simulink library "PowerFlowLib"  (R2016a)
settings: Solver=ode45  StartTime=0.0  StopTime=10.0  RelTol=1e-3
undefined symbols (not defined in the file or in its folder): Air, AirProp, C, F1, F2, Fanmap, Fld1, Fld2, Fluid, fueltankdata, HydProp, HydraulicLoad, IBFD_exc, L, LoadFluidProps, magnitude, MSSN, n_alghts, PumpProp, pwr_alghts, R_fd_exc, Rcore, Ts, VBFD_exc
libraries: PowerFlowLib x35, simulink x19, powerlib_extras x2, dspstat3 x2
(part 11 of 12)

== system PowerFlowLib/Energy & Power Systems/Thermal/ECS/Cabin Zone/Cabin Temperature ==
  Sup. Air Temp [C] : Inport
  Cabin mdot & mass : Inport  Port=2
  Cabin Param. : Inport  Port=3
  Air Props. : Inport  Port=4
  Amb Temp [K] : Inport  Port=5
  Mach # : Inport  Port=6
  Add : Sum  Inputs=+++
  Add1 : Sum  Inputs=+-+
  Bus Selector : BusSelector  OutputSignals=m_dot_sa,m_cab,m_dot_ra,m_dot_ea
  Bus Selector1 : BusSelector  OutputSignals=signal2.Cp_sa,signal1.Cp_cab,signal3.Cp_ra,signal4.Cp_ea
  Bus Selector2 : BusSelector  OutputSignals=n_pass,q_pass_W
  Bus Selector3 : BusSelector  OutputSignals=area_m2,U_Wpm2K
  Fuselage_parameters1 : Subsystem
  Integrator : Integrator  InitialCondition=20
  K_to_C : Bias  Bias=-273.15
  Kinetic Heating : Subsystem
  Scope : Scope
  Scope1 : Scope
  Scope2 : Scope  NumInputPorts=5
  adding_the_fuselage transmission_term_to the_const_term : Sum
  const_term fuselage_part : Product  Inputs=***//
  const_term pass_part : Product  Inputs=**//
  t_cab_term : Product  Inputs=**//
  t_cab_term_01 : Product  Inputs=**
  t_cab_term_02 : Product  Inputs=**
  t_cab_term_03 : Product  Inputs=**
  t_sa_term : Product  Inputs=***//
  Cabin Temp. [C] : Outport
  wires:
  K_to_C/1 -> const_term fuselage_part/3
  const_term fuselage_part/1 -> adding_the_fuselage transmission_term_to the_const_term/2
  adding_the_fuselage transmission_term_to the_const_term/1 -> Add1/3
  const_term pass_part/1 -> adding_the_fuselage transmission_term_to the_const_term/1
  t_cab_term_03/1 -> Add/3
  Bus Selector3/2 -> const_term fuselage_part/2, t_cab_term_03/2  "<U_Wpm2K>"
  Bus Selector3/1 -> const_term fuselage_part/1, t_cab_term_03/1  "<area_m2>"
  Fuselage_parameters1/1(Fuselage Parameters) -> Bus Selector3/1
  Integrator/1 -> Cabin Temp. [C]/1, t_cab_term/2
  Add1/1 -> Integrator/1  "dTcab/dt"
  Add/1 -> t_cab_term/1
  t_cab_term/1 -> Add1/2, Scope1/1
  t_sa_term/1 -> Add1/1, Scope/1
  t_cab_term_02/1 -> Add/2
  t_cab_term_01/1 -> Add/1
  Bus Selector1/4 -> t_cab_term_02/2  "<Cp_ea>"
  Bus Selector/4 -> t_cab_term_02/1  "<m_dot_ea>"
  Bus Selector1/3 -> t_cab_term_01/2  "<Cp_ra>"
  Bus Selector/3 -> t_cab_term_01/1  "<m_dot_ra>"
  Bus Selector2/2 -> const_term pass_part/2  "<q_pass_W>"
  Bus Selector2/1 -> const_term pass_part/1  "<n_pass>"
  Cabin Param./1 -> Bus Selector2/1
  Bus Selector1/2 -> t_cab_term/4, t_sa_term/5, Scope2/5, const_term pass_part/3, const_term fuselage_part/5  "<Cp_cab>"
  Bus Selector/2 -> t_cab_term/3, t_sa_term/4, Scope2/4, const_term pass_part/4, const_term fuselage_part/4  "<m_cab>"
  Bus Selector1/1 -> t_sa_term/3, Scope2/3  "<Cp_sa>"
  Bus Selector/1 -> t_sa_term/2, Scope2/2  "<m_dot_sa>"
  Sup. Air Temp [C]/1 -> t_sa_term/1, Scope2/1  "temp_sa_C"
  Air Props./1 -> Bus Selector1/1
  Cabin mdot & mass/1 -> Bus Selector/1
  Kinetic Heating/1(Recovery Temp [K]) -> K_to_C/1
  Mach #/1 -> Kinetic Heating/2(Mach#)
  Amb Temp [K]/1 -> Kinetic Heating/1(Amb. Temp. K)

== system PowerFlowLib/Energy & Power Systems/Thermal/ECS/Cabin Zone/Cabin_parameters ==
  note: Assuming that the thermal capacity of the cabin (C_p_cab)
      | is only due to the cabin air, not accounting for the furniture or
      | structure
  Bus Creator : BusCreator  Inputs=7
  Cp(P,T)3 : Lookup_n-D  BreakpointsForDimension1=AirProp.P  BreakpointsForDimension2=AirProp.T  BreakpointsForDimension3=[1]  Table=AirProp.Cp_pt  RndMeth=Simplest  InputSameDT=on
  Nominal cabin press_kPa : Constant  Value=80
  Nominal cabin temp_K : Constant  Value=298
  RAR : Constant  Value=RAR
  V_cab : Constant  Value=V_cab
  V_dot_sa_pass : Constant  Value=Vdot_sa_pass
  n_pack : Constant
  n_pass : Constant  Value=n_pass
  q_pass : Constant  Value=q_pass
  Cabin Parameters : Outport
  wires:
  Nominal cabin temp_K/1 -> Cp(P,T)3/2
  Nominal cabin press_kPa/1 -> Cp(P,T)3/1
  RAR/1 -> Bus Creator/7  "RAR"
  V_dot_sa_pass/1 -> Bus Creator/6  "V_dot_sa_pass"
  Bus Creator/1 -> Cabin Parameters/1
  Cp(P,T)3/1 -> Bus Creator/5  "C_p_cab_JKg^-1K^-1"
  n_pack/1 -> Bus Creator/4  "n_pack"
  q_pass/1 -> Bus Creator/3  "q_pass_W"
  V_cab/1 -> Bus Creator/2  "V_cab_m^3"
  n_pass/1 -> Bus Creator/1  "n_pass"

== system PowerFlowLib/Energy & Power Systems/Thermal/ECS/Cabin Zone/m_dot_sa_required1 ==
  Cabin Param. : Inport
  Sup. Air Prop. : Inport  Port=2
  Bus Selector : BusSelector  OutputSignals=n_pass,V_dot_sa_pass,n_pack
  Bus Selector1 : BusSelector  OutputSignals=Rho_sa
  Display : Display
  Display1 : Display
  Divide : Product  Inputs=***/
  mdot SA Req. : Outport
  wires:
  Divide/1 -> Display/1, mdot SA Req./1
  Bus Selector/3 -> Divide/4  "<n_pack>"
  Bus Selector1/1 -> Display1/1, Divide/3  "<Rho_sa>"
  Bus Selector/2 -> Divide/2  "<V_dot_sa_pass>"
  Bus Selector/1 -> Divide/1  "<n_pass>"
  Sup. Air Prop./1 -> Bus Selector1/1
  Cabin Param./1 -> Bus Selector/1

== system PowerFlowLib/Energy & Power Systems/Thermal/ECS/Fan/Air Properties ==
  Flow In : Inport
  Bus Creator : BusCreator  Inputs=2
  Bus Selector : BusSelector  OutputSignals=pres_kPa,temp_K
  Cp_in(P,T) : Lookup_n-D  BreakpointsForDimension1=AirProp.P  BreakpointsForDimension2=AirProp.T  BreakpointsForDimension3=[1]  Table=AirProp.Cp_pt  RndMeth=Simplest  InputSameDT=on
  Gain1 : Gain  Gain=1000
  Rho_in(P,T)1 : Lookup_n-D  BreakpointsForDimension1=AirProp.P  BreakpointsForDimension2=AirProp.T  BreakpointsForDimension3=[1]  Table=AirProp.Rho_pt  RndMeth=Simplest  InputSameDT=on
  AirProp : Outport
  wires:
  Bus Creator/1 -> AirProp/1
  Cp_in(P,T)/1 -> Gain1/1  "Cp_JpkgK"
  Rho_in(P,T)1/1 -> Bus Creator/1  "Rho_in_kgpm3"
  Bus Selector/2 -> Cp_in(P,T)/2, Rho_in(P,T)1/2  "<temp_K>"
  Bus Selector/1 -> Cp_in(P,T)/1, Rho_in(P,T)1/1  "<pres_kPa>"
  Flow In/1 -> Bus Selector/1
  Gain1/1 -> Bus Creator/2  "Cp_JpkgK"

== system PowerFlowLib/Energy & Power Systems/Thermal/ECS/Fan/Performance_curves_1725 rpm ==
  note: NOTE that the perfromance curves are given
      | at an air density of 1.2 kg/m3
  Vol_flow_rate_cfm_in : Inport
  in_flow_bus : Inport  Port=2
  Air_properties_at_inlet : Inport  Port=3
  Add : Sum
  Add1 : Sum  Inputs=+-
  Add2 : Sum
  BHP_1725 : Lookup_n-D  NumberOfTableDimensions=1  BreakpointsForDimension1=Fanmap.GH_SQ130_cfm_1725  Table=Fanmap.GH_SQ130_bhp_1725  RndMeth=Simplest  InputSameDT=on
  Bias : Bias  Bias=0.00001
  Bus Selector : BusSelector  OutputSignals=pres_Pa,mdot_kgps,temp_C
  Bus Selector1 : BusSelector  OutputSignals=Rho_in_kgpm3,Cp_JpkgK
  Electric HP_to_kW : Gain  Gain=746
  Static_press_inWG_1725 : Lookup_n-D  NumberOfTableDimensions=1  BreakpointsForDimension1=Fanmap.GH_SQ130_cfm_1725  Table=Fanmap.GH_SQ130_pstatic_1725  RndMeth=Simplest  InputSameDT=on
  Table_density_kgpm1 : Constant  Value=1.2
  Table_density_kgpm3 : Constant  Value=1.2
  calc_fan_ efficiency : Product  Inputs=*/
  calc_fan_ exit_temp : Product  Inputs=*//
  calc_fan_ hydr_power : Product  Inputs=**
  cfm_to_m3ps : Gain  Gain=1/2118.88
  correcting_fan_elec_ power_for_density_ratio : Product  Inputs=**/
  correcting_static_press_ for_density_ratio : Product  Inputs=**/
  inWG_to_Pa : Gain  Gain=248.84
  Power_required_W : Outport
  fan_efficiency : Outport  Port=2
  Pressure_out_Pa : Outport  Port=3
  Temp_out_C : Outport  Port=4
  mass_kgps : Outport  Port=5
  wires:
  [temp_C_in] -> Add2/2
  Bias/1 -> calc_fan_ exit_temp/3
  correcting_fan_elec_ power_for_density_ratio/1 -> [fan_elec_power_W], Power_required_W/1  "power_W"
  [Rho_kgpm3_in] -> correcting_fan_elec_ power_for_density_ratio/1
  Table_density_kgpm1/1 -> correcting_fan_elec_ power_for_density_ratio/3
  Electric HP_to_kW/1 -> correcting_fan_elec_ power_for_density_ratio/2  "power_W"
  Add/1 -> Pressure_out_Pa/1  "press_Pa"
  correcting_static_press_ for_density_ratio/1 -> [static_press_Pa], Add/2  "static_press_Pa"
  Bus Selector/1 -> [press_Pa_in]  "<pres_Pa>"
  [mdot_kgps_in] -> mass_kgps/1
  Add2/1 -> Temp_out_C/1  "temp_C"
  Bus Selector/3 -> [temp_C_in]  "<temp_C>"
  calc_fan_ exit_temp/1 -> Add2/1
  [mdot_kgps_in] -> Bias/1
  Bus Selector/2 -> [mdot_kgps_in]  "<mdot_kgps>"
  [Cp_JpkgK_in] -> calc_fan_ exit_temp/2
  Bus Selector1/2 -> [Cp_JpkgK_in]  "<Cp_JpkgK>"
  Add1/1 -> calc_fan_ exit_temp/1
  [fan_hydr_power_W] -> Add1/2
  [fan_elec_power_W] -> Add1/1
  calc_fan_ efficiency/1 -> fan_efficiency/1  "fan_eff"
  [fan_elec_power_W] -> calc_fan_ efficiency/2
  calc_fan_ hydr_power/1 -> [fan_hydr_power_W], calc_fan_ efficiency/1
  [static_press_Pa] -> calc_fan_ hydr_power/1
  cfm_to_m3ps/1 -> calc_fan_ hydr_power/2
  [vol_flow_rate_cfm_in] -> cfm_to_m3ps/1
  BHP_1725/1 -> Electric HP_to_kW/1
  [Rho_kgpm3_in] -> correcting_static_press_ for_density_ratio/1
  Table_density_kgpm3/1 -> correcting_static_press_ for_density_ratio/3
  Bus Selector1/1 -> [Rho_kgpm3_in]  "<Rho_in_kgpm3>"
  [press_Pa_in] -> Add/1
  inWG_to_Pa/1 -> correcting_static_press_ for_density_ratio/2
  in_flow_bus/1 -> Bus Selector/1
  Air_properties_at_inlet/1 -> Bus Selector1/1
  Static_press_inWG_1725/1 -> inWG_to_Pa/1  "press_inwg"
  Vol_flow_rate_cfm_in/1 -> [vol_flow_rate_cfm_in], BHP_1725/1, Static_press_inWG_1725/1

== system PowerFlowLib/Energy & Power Systems/Thermal/Fuel & Oil/Flow Junction/Liquid Enthalpy//Pressure Calcs ==
  Mdot_Out : Inport
  Hfluid : Inport  Port=2
  Pfluid : Inport  Port=3
  Mdot_In : Inport  Port=4
  H_In : Inport  Port=5
  Add1 : Sum  Inputs=-+
  Add2 : Sum  Inputs=-+
  Add3 : Sum
  Divide : Product  Inputs=*/
  Divide1 : Product
  Divide2 : Product  Inputs=*/
  Divide3 : Product  Inputs=*/
  Dot Product : DotProduct  InputSameDT=on  OutDataTypeStr=Inherit: Inherit via internal rule
  Gain : Gain  Gain=1/V
  Gain1 : Gain  Gain=1/V
  Gain2 : Gain  Gain=Bm
  Rho (p,h) : Lookup2D  RowIndex=F1.P  ColumnIndex=F1.H  Table=F1.Rho_ph  SaturateOnIntegerOverflow=on  InputSameDT=on
  Rho (p,h)1 : Lookup2D  RowIndex=F1.P  ColumnIndex=F1.H  Table=F1.Rho_ph  SaturateOnIntegerOverflow=on  InputSameDT=on
  Sum of Elements : Sum  Inputs=+
  Hdot : Outport
  Pdot : Outport  Port=2
  wires:
  Pfluid/1 -> [Pfluid], Rho (p,h)/1
  H_In/1 -> Dot Product/2
  Hfluid/1 -> [Hfluid], Divide1/2
  Add3/1 -> Hdot/1  "Hdot"
  Mdot_Out/1 -> Add2/1
  [Hfluid] -> Rho (p,h)/2
  [Hfluid] -> Rho (p,h)1/2
  [Pfluid] -> Rho (p,h)1/1
  Rho (p,h)/1 -> Divide2/2, Divide/2
  Add2/1 -> Gain/1
  Mdot_In/1 -> Sum of Elements/1, Dot Product/1
  Sum of Elements/1 -> Divide1/1, Add2/2
  Dot Product/1 -> Add1/2
  Divide1/1 -> Add1/1
  Divide/1 -> Gain2/1
  Add1/1 -> Gain1/1
  Rho (p,h)1/1 -> Divide3/2
  Divide2/1 -> Add3/1
  Divide3/1 -> Add3/2
  Gain1/1 -> Divide3/1
  Gain/1 -> Divide/1
  Gain2/1 -> Pdot/1, Divide2/1  "Pdot"

== system PowerFlowLib/Energy & Power Systems/Thermal/Fuel & Oil/Fluid Tank/Wall Heat Transfer ==
  vol_per : Inport
  wall_T : Inport  Port=2
  fluid_T : Inport  Port=3
  Enable : EnablePort
  Abs : Abs
  Demux : Demux  Outputs=2
  Divide : Product  Inputs=**
  Divide1 : Product  Inputs=**
  Sum : Sum  Inputs=+-
  Sum1 : Sum  Inputs=-+
  Walls 1 to n : Constant  Value=1:size(fueltankdata.leftwingtank,2)
  dry HTC : Gain  Gain=dryHTC
  total area : Bias  Bias=-[fueltankdata.leftwingtank(11,:)]
  volume_% : Lookup_n-D  BreakpointsForDimension1=linspace(0,1,11)  BreakpointsForDimension2=linspace(1,6,6)  Table=fueltankdata.leftwingtank  RndMeth=Simplest  InputSameDT=on
  wet HTC : Gain  Gain=wetHTC
  Qwall_wet : Outport
  Qwall_dry : Outport  Port=2
  wires:
  Abs/1 -> dry HTC/1
  dry HTC/1 -> Divide1/1
  Divide1/1 -> Qwall_dry/1
  Divide/1 -> Qwall_wet/1
  total area/1 -> Abs/1  "dry area"
  wet HTC/1 -> Divide/1
  Sum1/1 -> Divide1/2  "T_wall - T_ull"
  Sum/1 -> Divide/2  "T_wall - T_fuel"
  wall_T/1 -> Sum1/2, Sum/1
  Demux/2 -> Sum1/1  "ullage temp"
  Demux/1 -> Sum/2  "fuel temp"
  fluid_T/1 -> Demux/1
  volume_%/1 -> wet HTC/1, total area/1  "wet area"
  vol_per/1 -> volume_%/1
  Walls 1 to n/1 -> volume_%/2

== system PowerFlowLib/Energy & Power Systems/Thermal/Fuel & Oil/Fluid Tank/Warning msg ==
  time : Inport
  Trigger : TriggerPort  TriggerType=falling  VariantControl=Variant
  MATLAB Function : MATLAB Function  TreatAsAtomicUnit=on
  Terminator : Terminator
  wires:
  MATLAB Function/1(y) -> Terminator/1
  time/1 -> MATLAB Function/1(time)

== system PowerFlowLib/Energy & Power Systems/Electrical/Battery/BATTERY/SINGLE CELL VOLT OUT/CHARGE ==
  NET BTRY CT : Inport
  SOC : Inport  Port=2
  Add : Sum  Inputs=++++
  Divide : Product  Inputs=*/
  Divide1 : Product  Inputs=*/
  Divide2 : Product  Inputs=*/
  Gain3 : Gain  Gain=-1
  Product : Product  RndMeth=Zero
  Product4 : Product  RndMeth=Zero
  RCh : Subsystem
  RCm : Subsystem
  RCs : Subsystem
  Rseries_C : Fcn  Expr=0.051+0.2078*u-1.1148*u^2+2.1656*u^3-1.7766*u^4+0.5251*u^5
  Sum{,1..3} (4 alike) : Sum  Inputs=++|
  V_OC : Fcn  Expr=3+13.433*u-90.038*u^2+284.33*u^3-453.64*u^4+355.88*u^5-108.97*u^6
  square{,1..3} (4 alike) : Fcn  Expr=u^2
  TERMINAL V : Outport
  POWER LOSS : Outport  Port=2
  wires:
  V_OC/1 -> Sum/1
  SOC/1 -> V_OC/1, Rseries_C/1, RCm/1(SOC), RCh/1(SOC), RCs/1(SOC)
  Sum/1 -> Sum1/1
  Product/1 -> Sum/2
  Rseries_C/1 -> [Rseries_Charge], Product/2
  NET BTRY CT/1 -> Gain3/1, square/1
  RCs/1(Drop) -> Sum1/2, [Vs_Charge]
  Sum1/1 -> Sum2/1
  RCm/1(Drop) -> Sum2/2, [Vm_Charge]
  RCh/1(Drop) -> Sum3/2, [Vh_Charge]
  Sum2/1 -> Sum3/1
  Sum3/1 -> TERMINAL V/1
  Gain3/1 -> Product/1, RCm/2(current), RCh/2(current), RCs/2(current)
  square/1 -> Product4/1
  [Rseries_Charge] -> Product4/2
  [Vs_Charge] -> square1/1
  square1/1 -> Divide/1
  [Rs_Charge] -> Divide/2
  [Vm_Charge] -> square2/1
  square2/1 -> Divide1/1
  [Rm_Charge] -> Divide1/2
  [Vh_Charge] -> square3/1
  square3/1 -> Divide2/1
  [Rh_Charge] -> Divide2/2
  Product4/1 -> Add/1
  Divide/1 -> Add/2
  Divide1/1 -> Add/3
  Divide2/1 -> Add/4
  Add/1 -> POWER LOSS/1
  RCm/2(Rm_Charge) -> [Rm_Charge]
  RCh/2(Rh_Charge) -> [Rh_Charge]
  RCs/2(Rs_Charge) -> [Rs_Charge]

== system PowerFlowLib/Energy & Power Systems/Electrical/Battery/BATTERY/SINGLE CELL VOLT OUT/DISCHARGE ==
  NET BTRY CT : Inport
  SOC : Inport  Port=2
  Add : Sum  Inputs=++++
  Divide : Product  Inputs=*/
  Divide1 : Product  Inputs=*/
  Divide2 : Product  Inputs=*/
  Product : Product  RndMeth=Zero
  Product4 : Product  RndMeth=Zero
  RCh : Subsystem
  RCm : Subsystem
  RCs : Subsystem
  Rseries : Fcn  Expr=0.0482+0.144*u-0.4577*u^2+0.4965*u^3-0.1297*u^4-0.049*u^5
  Sum{,1..3} (4 alike) : Sum  Inputs=+-|
  V_OC : Fcn  Expr=3+13.433*u-90.038*u^2+284.33*u^3-453.64*u^4+355.88*u^5-108.97*u^6
  square{,1..3} (4 alike) : Fcn  Expr=u^2
  TERMINAL V : Outport
  POWER LOSS : Outport  Port=2
  wires:
  V_OC/1 -> Sum/1
  SOC/1 -> V_OC/1, RCs/1(SOC), RCh/1(SOC), RCm/1(SOC), Rseries/1
  Sum/1 -> Sum1/1
  Rseries/1 -> Product/2, [Rseries_Dchg]
  NET BTRY CT/1 -> square/1, Product/1, RCs/2(current), RCh/2(current), RCm/2(current1)
  RCs/1(Drop) -> [Vs_Dchg], Sum1/2
  Sum1/1 -> Sum2/1
  Sum2/1 -> Sum3/1
  Sum3/1 -> TERMINAL V/1
  square/1 -> Product4/1
  [Rseries_Dchg] -> Product4/2
  [Vs_Dchg] -> square1/1
  square1/1 -> Divide/1
  [Rs_Dchg] -> Divide/2
  [Vm_Dchg] -> square2/1
  square2/1 -> Divide1/1
  [Rm_Dchg] -> Divide1/2
  [Vh_Dchg] -> square3/1
  square3/1 -> Divide2/1
  [Rh_Dchg] -> Divide2/2
  Product4/1 -> Add/1
  Divide/1 -> Add/2
  Divide1/1 -> Add/3
  Divide2/1 -> Add/4
  Add/1 -> POWER LOSS/1
  RCs/2(Rs_Dchg) -> [Rs_Dchg]
  RCh/2(Rh_Dchg) -> [Rh_Dchg]
  RCh/1(Drop) -> [Vh_Dchg], Sum3/2
  Product/1 -> Sum/2
  RCm/1(Drop) -> Sum2/2, [Vm_Dchg]
  RCm/2(Rm_Dchg) -> [Rm_Dchg]

== system PowerFlowLib/Energy & Power Systems/Electrical/Battery/BATTERY/SOC /SOC _ DISCHARGE ==
  INTIAL SOC : Inport
  NET BTRY CT : Inport  Port=2
  1-D Lookup Table : Lookup_n-D  NumberOfTableDimensions=1  BreakpointsForDimension1=[0 0.0808 0.4389 1.0886 2.1603]  BreakpointsForDimension1DataTypeStr=Inherit: Inherit from 'Breakpoint data'  Table=[-1.4e-4 -1/(0.0808*3600*25) -1.00542/(0.4389*3600*5) -1.03632/(1.0886*2*3600) -1.08318/(2.1603*3600)]  RndMeth=Simplest  InputSameDT=on
  Integrator : Integrator
  Product : Product  RndMeth=Zero
  Saturation1 : Saturate  UpperLimit=1  LowerLimit=0
  Sum : Sum  Inputs=|++
  DYNAMIC SOC : Outport
  wires:
  Saturation1/1 -> DYNAMIC SOC/1
  NET BTRY CT/1 -> Product/1, 1-D Lookup Table/1
  Sum/1 -> Saturation1/1
  Integrator/1 -> Sum/2
  Product/1 -> Integrator/1
  1-D Lookup Table/1 -> Product/2
  INTIAL SOC/1 -> Sum/1

== system PowerFlowLib/Energy & Power Systems/Electrical/Battery/BATTERY/SOC /SOC_CHARGE ==
  INITIAL SOC : Inport
  NET BTRY CT : Inport  Port=2
  1-D Lookup Table2 : Lookup_n-D  NumberOfTableDimensions=1  BreakpointsForDimension1=[0 0.0838 0.4386 1.0988 2.202]  BreakpointsForDimension1DataTypeStr=Inherit: Inherit from 'Breakpoint data'  Table=[1.34e-4 1/(0.0838*3600*25) 0.99324/(0.4386*3600*5) 0.9803/(1.0988*2*3600) 0.98/(2.202*3600)]  RndMeth=Simplest  InputSameDT=on
  Gain : Gain  Gain=-1
  Integrator : Integrator
  Product : Product  RndMeth=Zero
  Sum : Sum  Inputs=|++
  DYNAMIC SOC : Outport
  wires:
  Gain/1 -> 1-D Lookup Table2/1, Product/1
  NET BTRY CT/1 -> Gain/1
  Sum/1 -> DYNAMIC SOC/1
  Integrator/1 -> Sum/2
  Product/1 -> Integrator/1
  1-D Lookup Table2/1 -> Product/2
  INITIAL SOC/1 -> Sum/1

== system PowerFlowLib/Energy & Power Systems/Electrical/Inverters/ Inverter/Three-Phase Full Bridge Inverter CONSTANT FREQUENCY1/Switch Loss ==
  Vdc : Inport
  Trise : Inport  Port=2
  Tfall : Inport  Port=3
  Inverter phase current : Inport  Port=4
  Fsw mean : Inport  Port=5
  Add : Sum
  Divide : Product  Inputs=****
  Gain : Gain  Gain=0.5
  Switch Loss : Outport
  wires:
  Vdc/1 -> Divide/1
  Trise/1 -> Add/1
  Tfall/1 -> Add/2
  Add/1 -> Gain/1
  Inverter phase current/1 -> Divide/3
  Fsw mean/1 -> Divide/4
  Divide/1 -> Switch Loss/1
  Gain/1 -> Divide/2

== system PowerFlowLib/Energy & Power Systems/Electrical/Inverters/1phs Inverter (2-level) - switching/2-level PWM/Tri(t) ==
  Clock : Clock
      settings: DisableCoverage=on
  Constant : Constant  DisableCoverage=on  Value=period
  Look-Up Table1 : Lookup  DisableCoverage=on  InputValues=rep_seq_t - min(rep_seq_t)  Table=rep_seq_y  SaturateOnIntegerOverflow=on
  Math Function : Math  DisableCoverage=on  Operator=rem  SaturateOnIntegerOverflow=on
  Output : SignalConversion  ConversionOutput=Contiguous copy  OverrideOpt=off
  Sum : Sum  DisableCoverage=on  Inputs=+-  SaturateOnIntegerOverflow=on  InputSameDT=on  OutDataTypeStr=Inherit: Same as first input
  startTime : S-Function  DisableCoverage=on  FunctionName=sfun_tstart  SFunctionDeploymentMode=off  EnableBusSupport=off
  Out1 : Outport
  wires:
  Math Function/1 -> Look-Up Table1/1
  Sum/1 -> Math Function/1
  Clock/1 -> Sum/1
  startTime/1 -> Sum/2
  Look-Up Table1/1 -> Output/1
  Output/1 -> Out1/1
  Constant/1 -> Math Function/2

== system PowerFlowLib/Energy & Power Systems/Electrical/Loads/Enabled_AC_Loadloss/Enabled Subsystem/CURRENT BASED LOADS ==
  note: SPLITTING CURRENT IN BOTH D AND Q AXES
  Constant : Constant  Value=0
  Constant1 : Constant  Value=ILRMS
  Gain1 : Gain  Gain=sqrt(2)
  Mux : Mux  Inputs=3
  Idqo : Outport
  wires:
  Constant1/1 -> Gain1/1
  Gain1/1 -> Mux/1, Mux/2
  Mux/1 -> Idqo/1
  Constant/1 -> Mux/3

== system PowerFlowLib/Energy & Power Systems/Electrical/Loads/Enabled_AC_Loadloss/Enabled Subsystem/IMPEDANCE BASED LOADS ==
  Vdq0 : Inport
  Constant1 : Constant  Value=R
  Constant2 : Constant  Value=X
  Constant3 : Constant  Value=R
  Constant4 : Constant  Value=X
  Demux : Demux  Outputs=3
  Fcn : Fcn  Expr=u(1)/(u(2)+0.1)
  Fcn1 : Fcn  Expr=u(1)/(u(2)+0.1)
  Math Function{,1..3} (4 alike) : Math  Operator=square  SaturateOnIntegerOverflow=on
  Mux : Mux  Inputs=3
  Mux1 : Mux  Inputs=2
  Mux2 : Mux  Inputs=2
  Product{1..2,5..6} (4 alike) : Product  Inputs=**  RndMeth=Zero
  Sum1 : Sum  Inputs=|++
  Sum2 : Sum  Inputs=|++
  Sum3 : Sum  Inputs=|+-
  Sum4 : Sum  Inputs=|++
  Idq0 : Outport
  wires:
  Mux/1 -> Idq0/1
  Mux2/1 -> Fcn1/1
  Mux1/1 -> Fcn/1
  Sum4/1 -> Mux2/2
  Sum3/1 -> Mux2/1
  Math Function3/1 -> Sum4/2
  Math Function2/1 -> Sum4/1
  Product6/1 -> Sum3/2
  Constant4/1 -> Math Function3/1, Product6/1
  Product5/1 -> Sum3/1
  Constant3/1 -> Math Function2/1, Product5/1
  Sum2/1 -> Mux1/2
  Math Function1/1 -> Sum2/2
  Math Function/1 -> Sum2/1
  Sum1/1 -> Mux1/1
  Product2/1 -> Sum1/2
  Constant2/1 -> Math Function1/1, Product2/1
  Demux/2 -> Product5/2, Product2/2
  Product1/1 -> Sum1/1
  Demux/1 -> Product6/2, Product1/2
  Constant1/1 -> Math Function/1, Product1/1
  Vdq0/1 -> Demux/1
  Fcn/1 -> Mux/1
  Fcn1/1 -> Mux/2

== system PowerFlowLib/Energy & Power Systems/Electrical/Loads/Enabled_AC_Loadloss/Enabled Subsystem/POWER BASED LOADS ==
  Vdq0 : Inport
  Constant1 : Constant  Value=P
  Constant2 : Constant  Value=PF
  Constant3 : Constant  Value=P
  Constant5 : Constant
  Constant6 : Constant  Value=0
  Constant7 : Constant  Value=P
  Demux : Demux  Outputs=3
  Fcn : Fcn  Expr=u(1)/(u(2)+0.1)
  Fcn1 : Fcn  Expr=u(1)/(u(2)+0.1)
  Math Function{,1..3} (4 alike) : Math  Operator=square  SaturateOnIntegerOverflow=on
  Mux : Mux  Inputs=3
  Mux1 : Mux  Inputs=2
  Mux2 : Mux  Inputs=2
  Product1 : Product  Inputs=***  RndMeth=Zero
  Product2 : Product  Inputs=**  RndMeth=Zero
  Product3 : Product  Inputs=**  RndMeth=Zero
  Product5 : Product  Inputs=***  RndMeth=Zero
  Product6 : Product  Inputs=**  RndMeth=Zero
  Sum1 : Sum  Inputs=|++
  Sum2 : Sum  Inputs=|++
  Sum3 : Sum  Inputs=|+-
  Sum4 : Sum  Inputs=|++
  Trigonometric Function : Trigonometry  Operator=acos
  Trigonometric Function1 : Trigonometry  Operator=tan
  Idq0 : Outport
  loss : Outport  Port=2
  wires:
  Constant7/1 -> Product3/2
  Trigonometric Function1/1 -> Product3/1
  Trigonometric Function/1 -> Trigonometric Function1/1
  Fcn1/1 -> Mux/2
  Fcn/1 -> Mux/1
  Vdq0/1 -> Demux/1
  Demux/1 -> Product1/2, Math Function/1, Product6/2, Math Function3/1
  Product1/1 -> Sum1/1
  Demux/2 -> Product2/2, Math Function1/1, Product5/2, Math Function2/1
  Constant2/1 -> Trigonometric Function/1
  Product2/1 -> Sum1/2
  Sum1/1 -> Mux1/1
  Math Function/1 -> Sum2/1
  Math Function1/1 -> Sum2/2
  Sum2/1 -> Mux1/2
  Constant3/1 -> Product5/1
  Product5/1 -> Sum3/1
  Product3/1 -> Product2/1, Product6/1
  Product6/1 -> Sum3/2
  Math Function2/1 -> Sum4/1
  Math Function3/1 -> Sum4/2
  Sum3/1 -> Mux2/1
  Sum4/1 -> Mux2/2
  Mux1/1 -> Fcn/1
  Mux2/1 -> Fcn1/1
  Mux/1 -> Idq0/1
  Constant5/1 -> Product1/3
  Constant6/1 -> Product5/3
  Constant1/1 -> loss/1, Product1/1

== system PowerFlowLib/Energy & Power Systems/Electrical/Loads/Enabled_AC_Loadloss/Enabled Subsystem1/CURRENT BASED LOADS ==
  note: SPLITTING CURRENT IN BOTH D AND Q AXES
  Iconst RMS : Inport
  Gain1 : Gain  Gain=sqrt(2)
  Mux : Mux  Inputs=3
  Idqo : Outport
  wires:
  Mux/1 -> Idqo/1
  Gain1/1 -> Mux/2, Mux/1
  Iconst RMS/1 -> Gain1/1

== system PowerFlowLib/Energy & Power Systems/Electrical/Loads/Enabled_AC_Loadloss/Enabled Subsystem1/POWER BASED LOADS ==
  Vdq0 : Inport
  P : Inport  Port=2
  Q : Inport  Port=3
  Demux : Demux  Outputs=3
  Fcn : Fcn  Expr=u(1)/(u(2)+0.1)
  Fcn1 : Fcn  Expr=u(1)/(u(2)+0.1)
  Math Function{,1..3} (4 alike) : Math  Operator=square  SaturateOnIntegerOverflow=on
  Mux : Mux  Inputs=3
  Mux1 : Mux  Inputs=2
  Mux2 : Mux  Inputs=2
  Product{1..2,5..6} (4 alike) : Product  Inputs=**  RndMeth=Zero
  Sum1 : Sum  Inputs=|++
  Sum2 : Sum  Inputs=|++
  Sum3 : Sum  Inputs=|+-
  Sum4 : Sum  Inputs=|++
  Idq0 : Outport
  wires:
  Fcn1/1 -> Mux/2
  Fcn/1 -> Mux/1
  Mux/1 -> Idq0/1
  Mux2/1 -> Fcn1/1
  Mux1/1 -> Fcn/1
  Sum4/1 -> Mux2/2
  Sum3/1 -> Mux2/1
  Math Function3/1 -> Sum4/2
  Math Function2/1 -> Sum4/1
  Product6/1 -> Sum3/2
  Product5/1 -> Sum3/1
  Sum2/1 -> Mux1/2
  Math Function1/1 -> Sum2/2
  Math Function/1 -> Sum2/1
  Sum1/1 -> Mux1/1
  Product2/1 -> Sum1/2
  Q/1 -> Product6/1, Product2/1
  Demux/2 -> Math Function2/1, Product5/2, Math Function1/1, Product2/2
  Product1/1 -> Sum1/1
  P/1 -> Product5/1, Product1/1
  Vdq0/1 -> Demux/1
  Demux/1 -> Math Function3/1, Product6/2, Product1/2, Math Function/1

== system PowerFlowLib/Energy & Power Systems/Electrical/Machines/Permanent Magnet Synchronous Generator1/Generator Power Loss1/Heat Trasnfer ==
  Tamb : Inport
  Ts : Inport  Port=2
  1/R_conv : Gain  Gain=1/R_conv_exciter
  Sum : Sum  Inputs=|+-
  Pdiss : Outport
  wires:
  1/R_conv/1 -> Pdiss/1
  Sum/1 -> 1/R_conv/1
  Tamb/1 -> Sum/2
  Ts/1 -> Sum/1

== system PowerFlowLib/Energy & Power Systems/Electrical/Machines/Synchronous Machine P.U. dq0/Generator Power Loss1/Heat Trasnfer ==
  Tamb : Inport
  Ts : Inport  Port=2
  1/R_conv : Gain  Gain=1/R_conv_gen
  Sum : Sum  Inputs=|+-
  Pdiss : Outport
  wires:
  1/R_conv/1 -> Pdiss/1
  Sum/1 -> 1/R_conv/1
  Tamb/1 -> Sum/2
  Ts/1 -> Sum/1

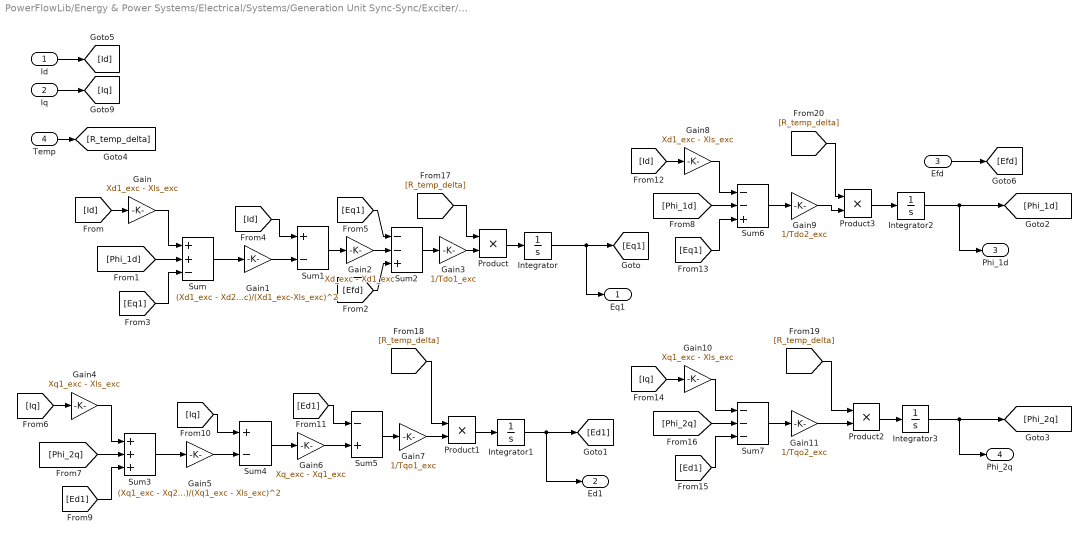
== system PowerFlowLib/Energy & Power Systems/Electrical/Systems/Generation Unit Sync-Sync/Exciter/Dynamics ==
  Id : Inport
  Iq : Inport  Port=2
  Efd : Inport  Port=3
  Temp : Inport  Port=4
  Gain : Gain  Gain=Xd1_exc - Xls_exc
  Gain1 : Gain  Gain=(Xd1_exc - Xd2_exc)/(Xd1_exc-Xls_exc)^2
  Gain10 : Gain  Gain=Xq1_exc - Xls_exc
  Gain11 : Gain  Gain=1/Tqo2_exc
  Gain2 : Gain  Gain=Xd_exc - Xd1_exc
  Gain3 : Gain  Gain=1/Tdo1_exc
  Gain4 : Gain  Gain=Xq1_exc - Xls_exc
  Gain5 : Gain  Gain=(Xq1_exc - Xq2_exc)/(Xq1_exc - Xls_exc)^2
  Gain6 : Gain  Gain=Xq_exc - Xq1_exc
  Gain7 : Gain  Gain=1/Tqo1_exc
  Gain8 : Gain  Gain=Xd1_exc - Xls_exc
  Gain9 : Gain  Gain=1/Tdo2_exc
  Integrator{,1..3} (4 alike) : Integrator
  Product{,1..3} (4 alike) : Product
  Sum : Sum  Inputs=++-
  Sum1 : Sum  Inputs=+-
  Sum2 : Sum  Inputs=--+
  Sum3 : Sum  Inputs=+++
  Sum4 : Sum  Inputs=+-
  Sum5 : Sum  Inputs=-+
  Sum6 : Sum  Inputs=--+
  Sum7 : Sum  Inputs=---
  Eq1 : Outport
  Ed1 : Outport  Port=2
  Phi_1d : Outport  Port=3
  Phi_2q : Outport  Port=4
  wires:
  Integrator/1 -> Eq1/1, [Eq1]
  [Id] -> Gain/1
  Gain/1 -> Sum/1
  [Phi_1d] -> Sum/2
  [Eq1] -> Sum/3
  Sum/1 -> Gain1/1
  [Id] -> Sum1/1
  Gain1/1 -> Sum1/2
  Sum1/1 -> Gain2/1
  [Eq1] -> Sum2/1
  Gain2/1 -> Sum2/2
  [Efd] -> Sum2/3
  Sum2/1 -> Gain3/1
  Integrator1/1 -> Ed1/1, [Ed1]
  [Iq] -> Gain4/1
  Gain4/1 -> Sum3/1
  [Phi_2q] -> Sum3/2
  [Ed1] -> Sum3/3
  Sum3/1 -> Gain5/1
  [Iq] -> Sum4/1
  Gain5/1 -> Sum4/2
  Sum4/1 -> Gain6/1
  [Ed1] -> Sum5/1
  Gain6/1 -> Sum5/2
  Sum5/1 -> Gain7/1
  [Id] -> Gain8/1
  Gain8/1 -> Sum6/1
  [Phi_1d] -> Sum6/2
  [Eq1] -> Sum6/3
  Sum6/1 -> Gain9/1
  Integrator2/1 -> [Phi_1d], Phi_1d/1
  [Iq] -> Gain10/1
  Gain10/1 -> Sum7/1
  [Phi_2q] -> Sum7/2
  [Ed1] -> Sum7/3
  Sum7/1 -> Gain11/1
  Integrator3/1 -> [Phi_2q], Phi_2q/1
  Id/1 -> [Id]
  Iq/1 -> [Iq]
  Efd/1 -> [Efd]
  Temp/1 -> [R_temp_delta]
  Gain3/1 -> Product/2
  Product/1 -> Integrator/1
  [R_temp_delta] -> Product/1
  [R_temp_delta] -> Product1/1
  Gain7/1 -> Product1/2
  Product1/1 -> Integrator1/1
  [R_temp_delta] -> Product2/1
  Gain11/1 -> Product2/2
  Product2/1 -> Integrator3/1
  [R_temp_delta] -> Product3/1
  Gain9/1 -> Product3/2
  Product3/1 -> Integrator2/1

== system PowerFlowLib/Energy & Power Systems/Electrical/Systems/Generation Unit Sync-Sync/Exciter/Electromagnetic Torque Output Power ==
  note: Torque from Field Winding
  note: Torque from Damper Windings
  Id : Inport
  Iq : Inport  Port=2
  Eq1 : Inport  Port=3
  Ed1 : Inport  Port=4
  Phi_1d : Inport  Port=5
  Phi_2q : Inport  Port=6
  Gain : Gain  Gain=(Xd2_exc - Xls_exc)/(Xd1_exc - Xls_exc)
  Gain1 : Gain  Gain=(Xq2_exc - Xls_exc)/(Xq1_exc - Xls_exc)
  Gain2 : Gain  Gain=(Xd1_exc - Xd2_exc)/(Xd1_exc-Xls_exc)
  Gain3 : Gain  Gain=(Xq1_exc - Xq2_exc)/(Xq1_exc-Xls_exc)
  Gain4 : Gain  Gain=(Xq2_exc - Xd2_exc)
  Product{,1..4} (5 alike) : Product  RndMeth=Zero
  Sum : Sum
  Sum1 : Sum  Inputs=+-+
  Sum2 : Sum
  TE : Outport
  wires:
  Id/1 -> [Id]
  Eq1/1 -> [Eq1]
  Ed1/1 -> [Ed1]
  Phi_1d/1 -> [Phi_1d]
  Phi_2q/1 -> [Phi_2q]
  Iq/1 -> [Iq]
  [Eq1] -> Product/1
  [Iq] -> Product/2
  Product/1 -> Gain/1
  [Ed1] -> Product1/1
  [Id] -> Product1/2
  Product1/1 -> Gain1/1
  [Iq] -> Product2/1
  [Phi_1d] -> Product2/2
  Product2/1 -> Gain2/1
  [Id] -> Product3/1
  [Phi_2q] -> Product3/2
  Product3/1 -> Gain3/1
  [Id] -> Product4/1
  [Iq] -> Product4/2
  Product4/1 -> Gain4/1
  Gain3/1 -> Sum1/2
  Gain2/1 -> Sum1/1
  Gain4/1 -> Sum1/3
  Gain/1 -> Sum/1
  Gain1/1 -> Sum/2
  Sum/1 -> Sum2/1
  Sum1/1 -> Sum2/2
  Sum2/1 -> TE/1

== system PowerFlowLib/Energy & Power Systems/Electrical/Systems/Generation Unit Sync-Sync/Exciter/Generator Power Loss ==
  Ed : Inport
  Eq : Inport  Port=2
  Id : Inport  Port=3
  Iq : Inport  Port=4
  Te : Inport  Port=5
  w/ws : Inport  Port=6
  Bus Creator : BusCreator  Inputs=6
  Gain1 : Gain  Gain=SB_exc
  Gain2 : Gain  Gain=SB_exc
  Gain3 : Gain  Gain=SB_exc
  Product : Product  RndMeth=Zero
  Product1 : Product  RndMeth=Zero
  Product2 : Product  RndMeth=Zero
  Sum1 : Sum  Inputs=-+
  Sum2 : Sum
  PE : Outport
  PM : Outport  Port=2
  PLOSS : Outport  Port=3
  m : Outport  Port=4
  wires:
  Ed/1 -> [Ed]
  Eq/1 -> [Eq]
  Id/1 -> [Id]
  Iq/1 -> [Iq]
  Te/1 -> [Te]
  w/ws/1 -> [nu]
  [Ed] -> Product/1
  [Id] -> Product/2
  [Eq] -> Product1/1
  [Iq] -> Product1/2
  [Te] -> Product2/1
  [nu] -> Product2/2
  Product/1 -> Sum2/1
  Product1/1 -> Sum2/2
  Sum2/1 -> Sum1/1, Gain1/1
  Product2/1 -> Sum1/2, Gain3/1
  Sum1/1 -> Gain2/1
  [Ed] -> Bus Creator/1  "Vd"
  [Id] -> Bus Creator/2  "Id"
  [Eq] -> Bus Creator/3  "Vq"
  [Iq] -> Bus Creator/4  "Iq"
  [Te] -> Bus Creator/5  "Te"
  [nu] -> Bus Creator/6  "nu"
  Bus Creator/1 -> m/1
  Gain2/1 -> PLOSS/1
  Gain1/1 -> PE/1
  Gain3/1 -> PM/1

== system PowerFlowLib/Energy & Power Systems/Electrical/Systems/Generation Unit Sync-Sync/Exciter/Stator Voltage ==
  Id : Inport
  Iq : Inport  Port=2
  Eq1 : Inport  Port=3
  Ed1 : Inport  Port=4
  Phi_1d : Inport  Port=5
  Phi_2q : Inport  Port=6
  w/ws : Inport  Port=7
  Temp : Inport  Port=8
  Gain : Gain  Gain=(Xq2_exc - Xls_exc)/(Xq1_exc - Xls_exc)
  Gain1 : Gain  Gain=(Xq1_exc - Xq2_exc)/(Xq1_exc - Xls_exc)
  Gain2 : Gain  Gain=(Xq2_exc - Xd2_exc)
  Gain3 : Gain  Gain=(Xd2_exc - Xls_exc)/(Xd1_exc - Xls_exc)
  Gain4 : Gain  Gain=(Xd1_exc - Xd2_exc)/(Xd1_exc - Xls_exc)
  Gain5 : Gain  Gain=Rs_exc
  Gain6 : Gain  Gain=Xd2+XTL
  Gain7 : Gain  Gain=Rs_exc+RTL_exc
  Gain8 : Gain  Gain=Xd2_exc+XTL_exc
  Product{,1..3,5} (5 alike) : Product  RndMeth=Zero
  Product4 : Product
  Sum : Sum
  Sum1 : Sum  Inputs=+-+
  Sum2 : Sum  Inputs=--+
  Sum3 : Sum  Inputs=-++
  Ed : Outport
  Eq : Outport  Port=2
  wires:
  Ed1/1 -> Gain/1
  Phi_2q/1 -> Gain1/1
  Iq/1 -> Product5/2, Gain6/1, Gain2/1
  Eq1/1 -> Gain3/1
  Phi_1d/1 -> Gain4/1
  Gain4/1 -> Sum/2
  Gain3/1 -> Sum/1
  Gain/1 -> Sum1/1
  Gain1/1 -> Sum1/2
  Sum/1 -> Product/1
  Sum1/1 -> Product1/1
  w/ws/1 -> Product1/2, Product/2, Product3/2, Product2/1
  Product/1 -> Sum2/3
  Id/1 -> Gain5/1, Gain8/1
  Gain6/1 -> Product2/2
  Gain8/1 -> Product3/1
  Product1/1 -> Sum3/2
  Gain2/1 -> Sum1/3
  Product2/1 -> Sum3/3
  Sum3/1 -> Ed/1  "Vd"
  Sum2/1 -> Eq/1  "Vq"
  Product3/1 -> Sum2/1
  Gain7/1 -> Sum2/2
  Product4/1 -> Sum3/1
  Gain5/1 -> Product4/1
  Temp/1 -> Product5/1, Product4/2
  Product5/1 -> Gain7/1

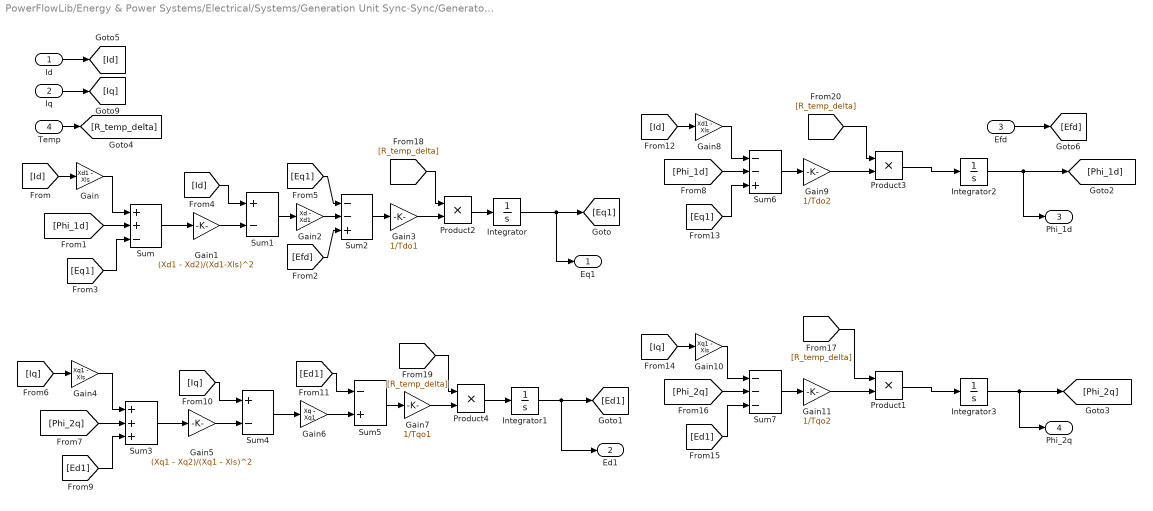
== system PowerFlowLib/Energy & Power Systems/Electrical/Systems/Generation Unit Sync-Sync/Generator/Dynamics ==
  Id : Inport
  Iq : Inport  Port=2
  Efd : Inport  Port=3
  Temp : Inport  Port=4
  Gain : Gain  Gain=Xd1 - Xls
  Gain1 : Gain  Gain=(Xd1 - Xd2)/(Xd1-Xls)^2
  Gain10 : Gain  Gain=Xq1 - Xls
  Gain11 : Gain  Gain=1/Tqo2
  Gain2 : Gain  Gain=Xd - Xd1
  Gain3 : Gain  Gain=1/Tdo1
  Gain4 : Gain  Gain=Xq1 - Xls
  Gain5 : Gain  Gain=(Xq1 - Xq2)/(Xq1 - Xls)^2
  Gain6 : Gain  Gain=Xq - Xq1
  Gain7 : Gain  Gain=1/Tqo1
  Gain8 : Gain  Gain=Xd1 - Xls
  Gain9 : Gain  Gain=1/Tdo2
  Integrator{,1..3} (4 alike) : Integrator
  Product{1..4} (4 alike) : Product
  Sum : Sum  Inputs=++-
  Sum1 : Sum  Inputs=+-
  Sum2 : Sum  Inputs=--+
  Sum3 : Sum  Inputs=+++
  Sum4 : Sum  Inputs=+-
  Sum5 : Sum  Inputs=-+
  Sum6 : Sum  Inputs=--+
  Sum7 : Sum  Inputs=---
  Eq1 : Outport
  Ed1 : Outport  Port=2
  Phi_1d : Outport  Port=3
  Phi_2q : Outport  Port=4
  wires:
  Efd/1 -> [Efd]
  Iq/1 -> [Iq]
  Id/1 -> [Id]
  Integrator3/1 -> Phi_2q/1, [Phi_2q]
  Sum7/1 -> Gain11/1
  [Ed1] -> Sum7/3
  [Phi_2q] -> Sum7/2
  Gain10/1 -> Sum7/1
  [Iq] -> Gain10/1
  Integrator2/1 -> Phi_1d/1, [Phi_1d]
  Sum6/1 -> Gain9/1
  [Eq1] -> Sum6/3
  [Phi_1d] -> Sum6/2
  Gain8/1 -> Sum6/1
  [Id] -> Gain8/1
  Sum5/1 -> Gain7/1
  Gain6/1 -> Sum5/2
  [Ed1] -> Sum5/1
  Sum4/1 -> Gain6/1
  Gain5/1 -> Sum4/2
  [Iq] -> Sum4/1
  Sum3/1 -> Gain5/1
  [Ed1] -> Sum3/3
  [Phi_2q] -> Sum3/2
  Gain4/1 -> Sum3/1
  [Iq] -> Gain4/1
  Integrator1/1 -> [Ed1], Ed1/1
  Sum2/1 -> Gain3/1
  [Efd] -> Sum2/3
  Gain2/1 -> Sum2/2
  [Eq1] -> Sum2/1
  Sum1/1 -> Gain2/1
  Gain1/1 -> Sum1/2
  [Id] -> Sum1/1
  Sum/1 -> Gain1/1
  [Eq1] -> Sum/3
  [Id] -> Gain/1
  Integrator/1 -> [Eq1], Eq1/1
  Gain/1 -> Sum/1
  [Phi_1d] -> Sum/2
  Temp/1 -> [R_temp_delta]
  [R_temp_delta] -> Product3/1
  Gain9/1 -> Product3/2
  Product3/1 -> Integrator2/1
  [R_temp_delta] -> Product1/1
  Gain11/1 -> Product1/2
  Product1/1 -> Integrator3/1
  [R_temp_delta] -> Product2/1
  Gain3/1 -> Product2/2
  Product2/1 -> Integrator/1
  [R_temp_delta] -> Product4/1
  Gain7/1 -> Product4/2
  Product4/1 -> Integrator1/1

== system PowerFlowLib/Energy & Power Systems/Electrical/Systems/Generation Unit Sync-Sync/Generator/Electromagnetic Torque Output Power ==
  note: Torque from Damper Windings
  note: Torque from Field Winding
  Id : Inport
  Iq : Inport  Port=2
  Eq1 : Inport  Port=3
  Ed1 : Inport  Port=4
  Phi_1d : Inport  Port=5
  Phi_2q : Inport  Port=6
  Gain : Gain  Gain=(Xd2 - Xls)/(Xd1 - Xls)
  Gain1 : Gain  Gain=(Xq2 - Xls)/(Xq1 - Xls)
  Gain2 : Gain  Gain=(Xd1 - Xd2)/(Xd1-Xls)
  Gain3 : Gain  Gain=(Xq1 - Xq2)/(Xq1-Xls)
  Gain4 : Gain  Gain=(Xq2 - Xd2)
  Product{,1..4} (5 alike) : Product  RndMeth=Zero
  Sum : Sum
  Sum1 : Sum  Inputs=+-+
  Sum2 : Sum
  TE : Outport
  wires:
  Sum2/1 -> TE/1
  Sum1/1 -> Sum2/2
  Sum/1 -> Sum2/1
  Gain1/1 -> Sum/2
  Gain/1 -> Sum/1
  Gain4/1 -> Sum1/3
  Gain2/1 -> Sum1/1
  Gain3/1 -> Sum1/2
  Product4/1 -> Gain4/1
  [Iq] -> Product4/2
  [Id] -> Product4/1
  Product3/1 -> Gain3/1
  [Phi_2q] -> Product3/2
  [Id] -> Product3/1
  Product2/1 -> Gain2/1
  [Phi_1d] -> Product2/2
  [Iq] -> Product2/1
  Product1/1 -> Gain1/1
  [Id] -> Product1/2
  [Ed1] -> Product1/1
  Product/1 -> Gain/1
  [Iq] -> Product/2
  [Eq1] -> Product/1
  Iq/1 -> [Iq]
  Phi_2q/1 -> [Phi_2q]
  Phi_1d/1 -> [Phi_1d]
  Ed1/1 -> [Ed1]
  Eq1/1 -> [Eq1]
  Id/1 -> [Id]

== system PowerFlowLib/Energy & Power Systems/Electrical/Systems/Generation Unit Sync-Sync/Generator/Generator Power Loss ==
  Ed : Inport
  Eq : Inport  Port=2
  Id : Inport  Port=3
  Iq : Inport  Port=4
  Te : Inport  Port=5
  w/ws : Inport  Port=6
  Bus Creator : BusCreator  Inputs=6
  Gain1 : Gain  Gain=SB
  Gain2 : Gain  Gain=SB
  Gain3 : Gain  Gain=SB
  Product : Product  RndMeth=Zero
  Product1 : Product  RndMeth=Zero
  Product2 : Product  RndMeth=Zero
  Sum1 : Sum  Inputs=-+
  Sum2 : Sum
  PE : Outport
  PM : Outport  Port=2
  PLOSS : Outport  Port=3
  m : Outport  Port=4
  wires:
  Gain3/1 -> PM/1
  Gain1/1 -> PE/1
  Gain2/1 -> PLOSS/1
  Bus Creator/1 -> m/1
  [nu] -> Bus Creator/6  "nu"
  [Te] -> Bus Creator/5  "Te"
  [Iq] -> Bus Creator/4  "Iq"
  [Eq] -> Bus Creator/3  "Vq"
  [Id] -> Bus Creator/2  "Id"
  [Ed] -> Bus Creator/1  "Vd"
  Sum1/1 -> Gain2/1
  Product2/1 -> Gain3/1, Sum1/2
  Sum2/1 -> Gain1/1, Sum1/1
  Product1/1 -> Sum2/2
  Product/1 -> Sum2/1
  [nu] -> Product2/2
  [Te] -> Product2/1
  [Iq] -> Product1/2
  [Eq] -> Product1/1
  [Id] -> Product/2
  [Ed] -> Product/1
  w/ws/1 -> [nu]
  Te/1 -> [Te]
  Iq/1 -> [Iq]
  Id/1 -> [Id]
  Eq/1 -> [Eq]
  Ed/1 -> [Ed]

== system PowerFlowLib/Energy & Power Systems/Electrical/Systems/Generation Unit Sync-Sync/Generator/Stator Voltage ==
  Id : Inport
  Iq : Inport  Port=2
  Eq1 : Inport  Port=3
  Ed1 : Inport  Port=4
  Phi_1d : Inport  Port=5
  Phi_2q : Inport  Port=6
  w/ws : Inport  Port=7
  Temp : Inport  Port=8
  Gain : Gain  Gain=(Xq2 - Xls)/(Xq1 - Xls)
  Gain1 : Gain  Gain=(Xq1 - Xq2)/(Xq1 - Xls)
  Gain2 : Gain  Gain=(Xq2 - Xd2)
  Gain3 : Gain  Gain=(Xd2 - Xls)/(Xd1 - Xls)
  Gain4 : Gain  Gain=(Xd1 - Xd2)/(Xd1 - Xls)
  Gain5 : Gain  Gain=Rs
  Gain6 : Gain  Gain=Xd2
  Gain7 : Gain  Gain=Rs
  Gain8 : Gain  Gain=Xd2
  Product{,1..3,5} (5 alike) : Product  RndMeth=Zero
  Product4 : Product
  Sum : Sum
  Sum1 : Sum  Inputs=+-+
  Sum2 : Sum  Inputs=--+
  Sum3 : Sum  Inputs=-++
  Ed : Outport
  Eq : Outport  Port=2
  wires:
  Gain7/1 -> Sum2/2
  Product3/1 -> Sum2/1
  Sum2/1 -> Eq/1  "Vq"
  Sum3/1 -> Ed/1  "Vd"
  Product2/1 -> Sum3/3
  Product1/1 -> Sum3/2
  Gain8/1 -> Product3/1
  Gain6/1 -> Product2/2
  Id/1 -> Gain8/1, Gain5/1
  Product/1 -> Sum2/3
  w/ws/1 -> Product2/1, Product3/2, Product/2, Product1/2
  Sum1/1 -> Product1/1
  Sum/1 -> Product/1
  Gain1/1 -> Sum1/2
  Gain/1 -> Sum1/1
  Gain3/1 -> Sum/1
  Gain4/1 -> Sum/2
  Phi_1d/1 -> Gain4/1
  Eq1/1 -> Gain3/1
  Phi_2q/1 -> Gain1/1
  Ed1/1 -> Gain/1
  Gain2/1 -> Sum1/3
  Temp/1 -> Product5/1, Product4/2
  Gain5/1 -> Product4/1
  Product4/1 -> Sum3/1
  Product5/1 -> Gain7/1
  Iq/1 -> Gain2/1, Product5/2, Gain6/1

== system PowerFlowLib/Energy & Power Systems/Electrical/Systems/three-phase full-bridge inverter/Three-Phase Full Bridge Inverter CONSTANT FREQUENCY1/Switch Loss ==
  Vdc : Inport
  Trise : Inport  Port=2
  Tfall : Inport  Port=3
  Inverter phase current : Inport  Port=4
  Fsw mean : Inport  Port=5
  Add : Sum
  Divide : Product  Inputs=****
  Gain : Gain  Gain=0.5
  Switch Loss : Outport
  wires:
  Gain/1 -> Divide/2
  Divide/1 -> Switch Loss/1
  Fsw mean/1 -> Divide/4
  Inverter phase current/1 -> Divide/3
  Add/1 -> Gain/1
  Tfall/1 -> Add/2
  Trise/1 -> Add/1
  Vdc/1 -> Divide/1

== system PowerFlowLib/Energy & Power Systems/Thermal/ECS/Air-Air HX/Air_properties_in_flows_hot_and_cold/air_properties_in_cold ==
  note: PLEASE NOTE that the air properties are based on the
      | inlet flow conditions rather than the average T and P.
      | Trying to base the properties on the average temperature
      | and even a constant pressure, the program did not work. One
      | suggestion is to average the inlet conditions with the outlet conditions
      | at a previous time step by using a memory block.x
  In_flow_bus_cold : Inport
  Bus Selector1 : BusSelector  OutputSignals=press_Pa,temp_C
  C to K : Bias  Bias=273
  Cp(P,T) : Lookup_n-D  BreakpointsForDimension1=AirProp.P  BreakpointsForDimension2=AirProp.T  BreakpointsForDimension3=[1]  Table=AirProp.Cp_pt  RndMeth=Simplest  InputSameDT=on
  Cp_pt_hot : Display
  Gain1 : Gain  Gain=1000
  Pa to kPa : Gain  Gain=10^-3
  Pr(P,T) : Lookup_n-D  BreakpointsForDimension1=AirProp.P  BreakpointsForDimension2=AirProp.T  BreakpointsForDimension3=[1]  Table=AirProp.Pr_pt  RndMeth=Simplest  InputSameDT=on
  Pr_pt_hot : Display
  Rho(P,T) : Lookup_n-D  BreakpointsForDimension1=AirProp.P  BreakpointsForDimension2=AirProp.T  BreakpointsForDimension3=[1]  Table=AirProp.Rho_pt  RndMeth=Simplest  InputSameDT=on
  Rho_pt_hot : Display
  k(P,T) : Lookup_n-D  BreakpointsForDimension1=AirProp.P  BreakpointsForDimension2=AirProp.T  BreakpointsForDimension3=[1]  Table=AirProp.k_pt  RndMeth=Simplest  InputSameDT=on
  k_pt_hot : Display
  mu(P,T) : Lookup_n-D  BreakpointsForDimension1=AirProp.P  BreakpointsForDimension2=AirProp.T  BreakpointsForDimension3=[1]  Table=AirProp.mu_pt  RndMeth=Simplest  InputSameDT=on
  mu_pt_hot : Display
  rho_air_kgm-3 : Outport
  cp_air_Jkg-1K-1 : Outport  Port=2
  mu_air_Pa.s : Outport  Port=3
  K_air_Wm-1K-2 : Outport  Port=4
  Pr : Outport  Port=5
  wires:
  In_flow_bus_cold/1 -> Bus Selector1/1
  C to K/1 -> Rho(P,T)/2, Pr(P,T)/2, k(P,T)/2, mu(P,T)/2, Cp(P,T)/2
  Bus Selector1/1 -> Pa to kPa/1  "<press_Pa>"
  Bus Selector1/2 -> C to K/1  "<temp_C>"
  Pa to kPa/1 -> Rho(P,T)/1, Cp(P,T)/1, mu(P,T)/1, Pr(P,T)/1, k(P,T)/1  "press_kPa"
  Rho(P,T)/1 -> Rho_pt_hot/1, rho_air_kgm-3/1
  Pr(P,T)/1 -> Pr_pt_hot/1, Pr/1
  k(P,T)/1 -> k_pt_hot/1, K_air_Wm-1K-2/1
  mu(P,T)/1 -> mu_pt_hot/1, mu_air_Pa.s/1
  Cp(P,T)/1 -> Cp_pt_hot/1, Gain1/1
  Gain1/1 -> cp_air_Jkg-1K-1/1

== system PowerFlowLib/Energy & Power Systems/Thermal/ECS/Air-Air HX/Air_properties_in_flows_hot_and_cold/air_properties_in_hot ==
  note: PLEASE NOTE that the air properties are based on the
      | inlet flow conditions rather than the average T and P.
      | Trying to base the properties on the average temperature
      | and even a constant pressure, the program did not work. One
      | suggestion is to average the inlet conditions with the outlet conditions
      | at a previous time step by using a memory block.x
  In_flow_bus_hot : Inport
  Bus Selector : BusSelector  OutputSignals=pres_Pa,temp_C
  C to K : Bias  Bias=273
  Cp(P,T) : Lookup_n-D  BreakpointsForDimension1=AirProp.P  BreakpointsForDimension2=AirProp.T  BreakpointsForDimension3=[1]  Table=AirProp.Cp_pt  RndMeth=Simplest  InputSameDT=on
  Cp_pt_hot : Display
  Gain : Gain  Gain=1000
  Pa to kPa : Gain  Gain=10^-3
  Pr(P,T) : Lookup_n-D  BreakpointsForDimension1=AirProp.P  BreakpointsForDimension2=AirProp.T  BreakpointsForDimension3=[1]  Table=AirProp.Pr_pt  RndMeth=Simplest  InputSameDT=on
  Pr_pt_hot : Display
  Rho(P,T) : Lookup_n-D  BreakpointsForDimension1=AirProp.P  BreakpointsForDimension2=AirProp.T  BreakpointsForDimension3=[1]  Table=AirProp.Rho_pt  RndMeth=Simplest  InputSameDT=on
  Rho_pt_hot : Display
  k(P,T) : Lookup_n-D  BreakpointsForDimension1=AirProp.P  BreakpointsForDimension2=AirProp.T  BreakpointsForDimension3=[1]  Table=AirProp.k_pt  RndMeth=Simplest  InputSameDT=on
  k_pt_hot : Display
  mu(P,T) : Lookup_n-D  BreakpointsForDimension1=AirProp.P  BreakpointsForDimension2=AirProp.T  BreakpointsForDimension3=[1]  Table=AirProp.mu_pt  RndMeth=Simplest  InputSameDT=on
  mu_pt_hot : Display
  rho_air_kgm-3 : Outport
  cp_air_Jkg-1K-1 : Outport  Port=2
  mu_air_Pa.s : Outport  Port=3
  K_air_Wm-1K-2 : Outport  Port=4
  Pr : Outport  Port=5
  wires:
  In_flow_bus_hot/1 -> Bus Selector/1
  C to K/1 -> Rho(P,T)/2, Pr(P,T)/2, k(P,T)/2, mu(P,T)/2, Cp(P,T)/2
  Bus Selector/1 -> Pa to kPa/1  "<pres_Pa>"
  Bus Selector/2 -> C to K/1  "<temp_C>"
  Pa to kPa/1 -> Rho(P,T)/1, Cp(P,T)/1, mu(P,T)/1, Pr(P,T)/1, k(P,T)/1  "press_kPa"
  Rho(P,T)/1 -> Rho_pt_hot/1, rho_air_kgm-3/1
  Pr(P,T)/1 -> Pr/1, Pr_pt_hot/1
  k(P,T)/1 -> K_air_Wm-1K-2/1, k_pt_hot/1
  mu(P,T)/1 -> mu_air_Pa.s/1, mu_pt_hot/1
  Cp(P,T)/1 -> Gain/1, Cp_pt_hot/1
  Gain/1 -> cp_air_Jkg-1K-1/1

== system PowerFlowLib/Energy & Power Systems/Thermal/ECS/Air-Air HX/HX_and_Fin_paramters/Fin_parameters ==
  Constant : Constant  Value=l_fin
  Constant1 : Constant  Value=t_fin
  Constant2 : Constant  Value=s_fin
  Constant3 : Constant  Value=h_fin
  Constant4 : Constant  Value=K_n
  Constant5 : Constant  Value=eta_f
  Fin_length_m : Outport
  Fin_thickness_m : Outport  Port=2
  Fin_free_flow_width_m : Outport  Port=3
  Fin_free_flow_height_m : Outport  Port=4
  K_fin_Wm-1K-1 : Outport  Port=5
  Fin_eff : Outport  Port=6
  wires:
  Constant1/1 -> Fin_thickness_m/1
  Constant2/1 -> Fin_free_flow_width_m/1
  Constant3/1 -> Fin_free_flow_height_m/1
  Constant4/1 -> K_fin_Wm-1K-1/1
  Constant5/1 -> Fin_eff/1
  Constant/1 -> Fin_length_m/1

== system PowerFlowLib/Energy & Power Systems/Thermal/ECS/Air-Air HX/HX_and_Fin_paramters/HX_parameters ==
  Other_HX_parameters : Inport
  Fin_parameters : Inport  Port=2
  Bus Selector : BusSelector  OutputSignals=L_hx
  Calculating the no of passages per fluid flow : Subsystem
  Calculating the total number of fins per HX per fluid flow : Subsystem
  Calculating total free flow area per flow : Subsystem
  Constant3 : Constant  Value=K_p
  Constant4 : Constant  Value=cp_hx
  Constant5 : Constant  Value=m_cm
  Display : Display
  Display1 : Display
  Display2 : Display
  tot_free_flow_area_m^2 : Outport
  tot_length_in_direc_of_flow_m : Outport  Port=2
  tot_no_of_fins_per_HX_per_flow : Outport  Port=3
  K_hx_Wm-1K-1 : Outport  Port=4
  cp_hx_Jkg-1K-1 : Outport  Port=5
  m_hx_kg : Outport  Port=6
  wires:
  Bus Selector/1 -> tot_length_in_direc_of_flow_m/1  "<L_hx>"
  Calculating the total number of fins per HX per fluid flow/1(Tot_no_of_fins_per_HX_per_flow) -> Display2/1, tot_no_of_fins_per_HX_per_flow/1  "N_f"
  Calculating total free flow area per flow/1(Total_free_flow_area) -> Display/1, tot_free_flow_area_m^2/1  "A"
  Calculating the no of passages per fluid flow/1(N_passages_per_flow) -> Display1/1, Calculating the total number of fins per HX per fluid flow/3(N_passages_per_flow), Calculating total free flow area per flow/3(N_passages_per_flow)
  Fin_parameters/1 -> Calculating the total number of fins per HX per fluid flow/2(Fin_parameters), Calculating total free flow area per flow/2(Fin_parameters), Calculating the no of passages per fluid flow/2(Fin_parameters)
  Other_HX_parameters/1 -> Bus Selector/1, Calculating the total number of fins per HX per fluid flow/1(Raw_HX_parameters), Calculating total free flow area per flow/1(Raw_HX_parameters), Calculating the no of passages per fluid flow/1(Raw_HX_parameters)
  Constant5/1 -> m_hx_kg/1
  Constant3/1 -> K_hx_Wm-1K-1/1
  Constant4/1 -> cp_hx_Jkg-1K-1/1

== system PowerFlowLib/Energy & Power Systems/Thermal/ECS/Air-Air HX/HX_and_Fin_paramters/Other_HX_parameters2 ==
  Bus Creator : BusCreator  Inputs=4
  Length in flow direction : Constant  Value=L_hx
  plate thickness : Constant  Value=t_p
  total height : Constant  Value=H_hx
  width : Constant  Value=W_hx
  Out1 : Outport
  wires:
  Bus Creator/1 -> Out1/1
  plate thickness/1 -> Bus Creator/4  "t_p"
  total height/1 -> Bus Creator/3  "H_hx"
  width/1 -> Bus Creator/2  "W_hx"
  Length in flow direction/1 -> Bus Creator/1  "L_hx"

== system PowerFlowLib/Energy & Power Systems/Thermal/ECS/Cabin Zone/Cabin Temperature/Fuselage_parameters1 ==
  Area_fuselage_total_m2 : Constant  Value=A_fuselage
  Bus Creator : BusCreator  Inputs=2
  Coating_resistance_ m2KpW : Product  Inputs=*/
  Coating_thermal_ conductivity_WpmK : Constant  Value=K_coating
  Coating_thickness_m : Constant  Value=L_coating
  Display : Display
  Inside_HTC_Wpm2K : Constant  Value=h_inside
  Inside_convection_ resistance_m2KpW : Product  Inputs=*/
  Insulation_resistance_ m2KpW : Product  Inputs=*/
  Insulation_thermal_ conductivity_WpmK : Constant  Value=K_insulation
  Insulation_thickness_m : Constant  Value=L_insulation
  Outside_HTC_Wpm2K1 : Constant  Value=h_outside
  Outside_convection_ resistance_m2KpW : Product  Inputs=*/
  Overall_HTC_based_on_ any_fuselage_area_Wpm2K : Product  Inputs=*/
  Shell_resistance_ m2KpW : Product  Inputs=*/
  Shell_thermal_ conductivity_WpmK : Constant  Value=K_shell
  Shell_thickness_m : Constant  Value=L_shell
  Total_resistance_ m2KpW : Sum  Inputs=+++++
  constant_unity : Constant
  constant_unity1 : Constant
  constant_unity2 : Constant
  Fuselage Parameters : Outport
  wires:
  Area_fuselage_total_m2/1 -> Bus Creator/1  "area_m2"
  Total_resistance_ m2KpW/1 -> Overall_HTC_based_on_ any_fuselage_area_Wpm2K/2
  constant_unity2/1 -> Overall_HTC_based_on_ any_fuselage_area_Wpm2K/1
  Inside_convection_ resistance_m2KpW/1 -> Total_resistance_ m2KpW/5
  Coating_resistance_ m2KpW/1 -> Total_resistance_ m2KpW/4
  Insulation_resistance_ m2KpW/1 -> Total_resistance_ m2KpW/3
  Shell_resistance_ m2KpW/1 -> Total_resistance_ m2KpW/2
  Outside_convection_ resistance_m2KpW/1 -> Total_resistance_ m2KpW/1
  Inside_HTC_Wpm2K/1 -> Inside_convection_ resistance_m2KpW/2
  constant_unity1/1 -> Inside_convection_ resistance_m2KpW/1
  Coating_thermal_ conductivity_WpmK/1 -> Coating_resistance_ m2KpW/2
  Coating_thickness_m/1 -> Coating_resistance_ m2KpW/1
  Insulation_thermal_ conductivity_WpmK/1 -> Insulation_resistance_ m2KpW/2
  Insulation_thickness_m/1 -> Insulation_resistance_ m2KpW/1
  Shell_thermal_ conductivity_WpmK/1 -> Shell_resistance_ m2KpW/2
  Shell_thickness_m/1 -> Shell_resistance_ m2KpW/1
  Outside_HTC_Wpm2K1/1 -> Outside_convection_ resistance_m2KpW/2
  constant_unity/1 -> Outside_convection_ resistance_m2KpW/1
  Bus Creator/1 -> Fuselage Parameters/1
  Overall_HTC_based_on_ any_fuselage_area_Wpm2K/1 -> Display/1, Bus Creator/2  "U_Wpm2K"

== system PowerFlowLib/Energy & Power Systems/Thermal/ECS/Cabin Zone/Cabin Temperature/Kinetic Heating ==
  note: PLEASE note that that the correlation for the recovery temperature
      | is gives in "Aircraft Systems", by Ian Moir and Allan Seabridge,
      | 3rd edition, pp 260
  Amb. Temp. K : Inport
  Mach# : Inport  Port=2
  Bias : Bias  Bias=1
  Gain : Gain  Gain=0.18
  Math Function1 : Math  Operator=magnitude^2  SaturateOnIntegerOverflow=on
  Product1 : Product  RndMeth=Zero
  Recovery Temp [K] : Outport
  wires:
  Math Function1/1 -> Gain/1
  Gain/1 -> Bias/1
  Bias/1 -> Product1/2
  Amb. Temp. K/1 -> Product1/1
  Product1/1 -> Recovery Temp [K]/1
  Mach#/1 -> Math Function1/1
